simulink model "hibrido_sim"  (R2013a)
settings: Solver=ode3  StartTime=0.0  StopTime=6  FixedStep=Tm  MaxStep=1e-2  RelTol=1e-3
values from neighbouring files (symbols this model uses):
  Ke = 1000    [fuerzas_var.m]    (also in hibrido_var.m)
  Kp = (2*pi*5)^2*eye(3)    [cartesiano_var.m]    (also in hibrido_var.m)
  Kpf = (2*pi*20)^2*eye(3)    [fuerzas_var.m]    (also in hibrido_var.m)
  Kv = 2*sqrt(Kp)*eye(3)    [cartesiano_var.m]    (also in hibrido_var.m)
  Kvf = 2*sqrt(Kpf)*eye(3)    [fuerzas_var.m]    (also in hibrido_var.m)
  q0 = [pi;1/4*pi]    [cartesiano_var.m]    (also in fuerzas_var.m = [0;pi/2]; hibrido_var.m = [0;pi/2])
  R0c = [cX0,cY0,cZ0]    [hibrido_var.m]
  robotTP = robotRR    [cartesiano_var.m]    (also in fuerzas_var.m; hibrido_var.m)
  Sfue = [zeros(1,3);[0,1,0];zeros(1,3)]    [hibrido_var.m]
  Spos = [[1,0,0];zeros(2,3)]    [hibrido_var.m]
  T0c = [R0c,cP0;[0,0,0,1]]    [hibrido_var.m]
undefined symbols (not defined in the file or in its folder): jacob0, modelAlpha, modelBeta
undefined symbols (not defined in the file): robotPlanta
libraries: roblocks x4
settings Model: Creator=Nicola  LastModifiedBy=Nicola

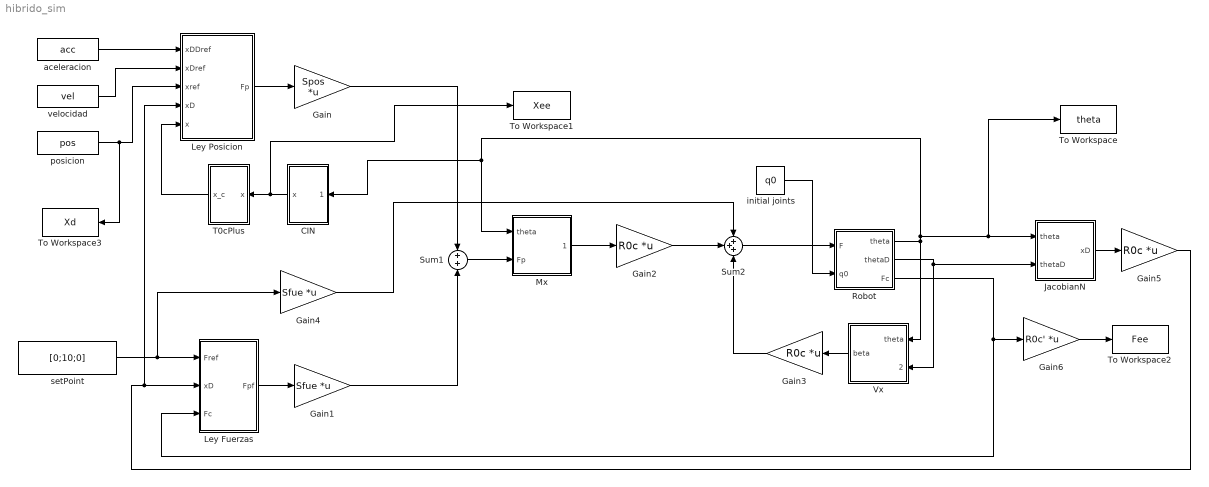
== system hibrido_sim ==
  CIN : Subsystem
  Gain : Gain  Gain=Spos  Multiplication=Matrix(K*u)
  Gain1 : Gain  Gain=Sfue  Multiplication=Matrix(K*u)
  Gain2 : Gain  Gain=R0c  Multiplication=Matrix(K*u)
  Gain3 : Gain  Gain=R0c  Multiplication=Matrix(K*u)
  Gain4 : Gain  Gain=Sfue  Multiplication=Matrix(K*u)
  Gain5 : Gain  Gain=R0c  Multiplication=Matrix(K*u)
  Gain6 : Gain  Gain=R0c'  Multiplication=Matrix(K*u)
  JacobianN : Subsystem
  Ley Fuerzas : Subsystem
  Ley Posicion : Subsystem
  Mx : Subsystem
  Robot : Subsystem
  Sum1 : Sum  Inputs=+|+
  Sum2 : Sum  Inputs=+++
  T0cPlus : Subsystem
  To Workspace : ToWorkspace  VariableName=theta  SampleTime=-1  SaveFormat=Timeseries
  To Workspace1 : ToWorkspace  VariableName=Xee  SampleTime=-1  SaveFormat=Timeseries
  To Workspace2 : ToWorkspace  VariableName=Fee  SampleTime=-1  SaveFormat=Timeseries
  To Workspace3 : ToWorkspace  VariableName=Xd  SampleTime=-1  SaveFormat=Timeseries
  Vx : Subsystem
  aceleracion : FromWorkspace  VariableName=acc  SampleTime=0
  initial joints : Constant  Value=q0
  posicion : FromWorkspace  VariableName=pos  SampleTime=0
  setPoint : Constant  Value=[0;10;0]
  velocidad : FromWorkspace  VariableName=vel  SampleTime=0
  wires:
  aceleracion/1 -> Ley Posicion/1(xDDref)
  velocidad/1 -> Ley Posicion/2(xDref)
  posicion/1 -> To Workspace3/1, Ley Posicion/3(xref)
  Ley Posicion/1(Fp) -> Gain/1
  Gain/1 -> Sum1/1
  setPoint/1 -> Gain4/1, Ley Fuerzas/1(Fref)
  Ley Fuerzas/1(Fpf) -> Gain1/1
  Gain1/1 -> Sum1/2
  Sum1/1 -> Mx/2(Fp)
  Mx/1(Mx*Fp) -> Gain2/1
  Vx/1(beta) -> Gain3/1
  Gain2/1 -> Sum2/2
  Gain3/1 -> Sum2/3
  Gain4/1 -> Sum2/1
  initial joints/1 -> Robot/2(q0)
  Sum2/1 -> Robot/1(F)
  Robot/1(theta) -> Vx/1(theta), To Workspace/1, JacobianN/1(theta), Mx/1(theta), CIN/1(theta)
  Robot/2(thetaD) -> Vx/2(thetaD), JacobianN/2(thetaD)
  Robot/3(Fc) -> Gain6/1, Ley Fuerzas/3(Fc)
  JacobianN/1(xD) -> Gain5/1
  Gain5/1 -> Ley Posicion/4(xD), Ley Fuerzas/2(xD)
  T0cPlus/1(x_c) -> Ley Posicion/5(x)
  CIN/1(x) -> To Workspace1/1, T0cPlus/1(x)
  Gain6/1 -> To Workspace2/1

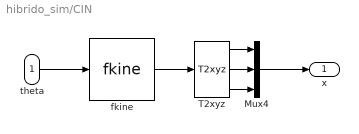
== system hibrido_sim/CIN ==
  theta : Inport
  Mux4 : Mux  Inputs=3
  T2xyz : roblocks/Transform Conversion/T2xyz
  fkine : roblocks/Kinematics/fkine  robot=robotTP.links
  x : Outport
  wires:
  T2xyz/1 -> Mux4/1
  T2xyz/3 -> Mux4/3
  Mux4/1 -> x/1
  T2xyz/2 -> Mux4/2
  theta/1 -> fkine/1
  fkine/1 -> T2xyz/1

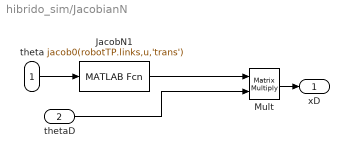
== system hibrido_sim/JacobianN ==
  theta : Inport
  thetaD : Inport  Port=2
  JacobN1 : MATLABFcn  MATLABFcn=jacob0(robotTP.links,u,'trans')  OutputDimensions=[3,2]  Output1D=off
  Mult : Product  Multiplication=Matrix(*)
  xD : Outport
  wires:
  Mult/1 -> xD/1
  thetaD/1 -> Mult/2
  JacobN1/1 -> Mult/1
  theta/1 -> JacobN1/1

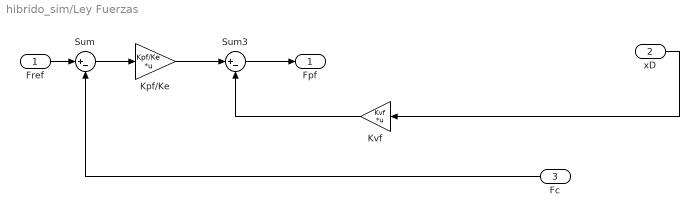
== system hibrido_sim/Ley Fuerzas ==
  Fref : Inport
  xD : Inport  Port=2
  Fc : Inport  Port=3
  Kpf/Ke : Gain  Gain=Kpf/Ke  Multiplication=Matrix(K*u)
  Kvf : Gain  Gain=Kvf  Multiplication=Matrix(K*u)
  Sum : Sum  Inputs=|+-
  Sum3 : Sum  Inputs=|+-
  Fpf : Outport
  wires:
  Fc/1 -> Sum/2
  Sum3/1 -> Fpf/1
  Sum/1 -> Kpf/Ke/1
  Kvf/1 -> Sum3/2
  Kpf/Ke/1 -> Sum3/1
  xD/1 -> Kvf/1
  Fref/1 -> Sum/1

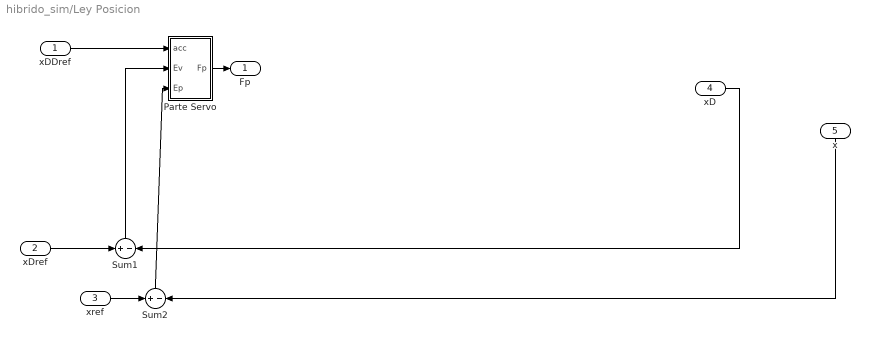
== system hibrido_sim/Ley Posicion ==
  xDDref : Inport
  xDref : Inport  Port=2
  xref : Inport  Port=3
  xD : Inport  Port=4
  x : Inport  Port=5
  Parte Servo : Subsystem
  Sum1 : Sum  Inputs=+|-
  Sum2 : Sum  Inputs=+|-
  Fp : Outport
  wires:
  xDDref/1 -> Parte Servo/1(acc)
  xDref/1 -> Sum1/1
  x/1 -> Sum2/2
  Parte Servo/1(Fp) -> Fp/1
  xref/1 -> Sum2/1
  Sum2/1 -> Parte Servo/3(Ep)
  Sum1/1 -> Parte Servo/2(Ev)
  xD/1 -> Sum1/2

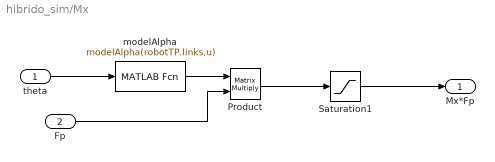
== system hibrido_sim/Mx ==
  theta : Inport
  Fp : Inport  Port=2
  Product : Product  Multiplication=Matrix(*)
  Saturation1 : Saturate  UpperLimit=1e10  LowerLimit=-1e10
  modelAlpha : MATLABFcn  MATLABFcn=modelAlpha(robotTP.links,u)  OutputDimensions=[3,3]  Output1D=off
  Mx*Fp : Outport
  wires:
  modelAlpha/1 -> Product/1
  Fp/1 -> Product/2
  theta/1 -> modelAlpha/1
  Product/1 -> Saturation1/1
  Saturation1/1 -> Mx*Fp/1

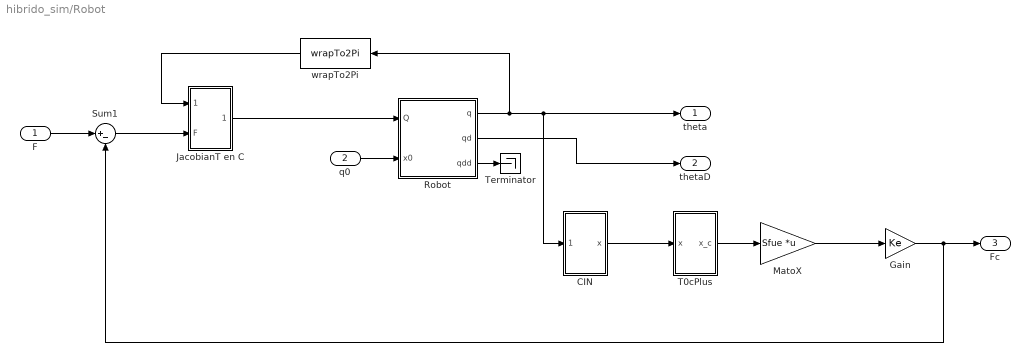
== system hibrido_sim/Robot ==
  F : Inport
  q0 : Inport  Port=2
  CIN : Subsystem
  Gain : Gain  Gain=Ke
  JacobianT en C : Subsystem
  MatoX : Gain  Gain=Sfue  Multiplication=Matrix(K*u)
  Robot : Subsystem  AncestorBlock=roblocks/Dynamics/Robot  mask{robot=robotPlanta, q0=[0,0,0,0,0,0]}
      mask prompts: robot "Robot object"; q0 "Initial state"
      mask help: Rigid-body dynamic model of robot.
      mask init:
      | if isa(robot, 'SerialLink')
      |     rname = robot.name;
      |     %fprintf('**robot name is %s\n', rname);
      | else
      |     rname = '';
      |     n = 0
      | end
      mask Help:
      | Simulates the forward (direct) rigid-body dynamics of the robot described
      | by the given robot object.  For given applied joint torque/force it computes
      | the instaneous joint coordinates, velocities and acclerations.
      | 
      | 
      | <b>Parameters::</b>
      | 
      | robot (SerialLink) a dynamic model of an N-link serial link manipulator
      | q0 (1xN)  Initial joint coordinates
      | 
      | <b>Inputs::</b>
      | 
      | Q (1xN) the generalized joint force (torque or force) required to achieve
      | the motion state (q, qd, qdd).
      | 
      | <b>Outputs::</b>
      | 
      | q (1xN) joint coordinates
      | qd (1xN) joint coordinate velocity
      | qdd (1xN) joint coordinate acceleration
      | 
      | 
      | <b>Notes::</b>
      | 
      | - Required to simulate robot rigid body motion.
      | - Implemented using the recursive Newton-Euler scheme (RNE).
      | - A wrapper for the Toolbox method accel() which in turn depends on the
      |   method rne().
      mask Display:
      | port_label('input', 1, 'Q')
      | port_label('output', 1, 'q')
      | port_label('output', 2, 'qd')
      | port_label('output', 3, 'qdd')
      | text(0.1, 0.9,  rname, 'horizontalAlignment', 'left')
  Sum1 : Sum  Inputs=|+-
  T0cPlus : Subsystem
  Terminator : Terminator
  wrapTo2Pi : MATLABFcn  MATLABFcn=wrapTo2Pi
  theta : Outport
  thetaD : Outport  Port=2
  Fc : Outport  Port=3
  wires:
  Robot/1(q) -> wrapTo2Pi/1, CIN/1(theta), theta/1
  Robot/3(qdd) -> Terminator/1
  Robot/2(qd) -> thetaD/1
  q0/1 -> Robot/2(x0)
  Gain/1 -> Sum1/2, Fc/1
  Sum1/1 -> JacobianT en C/2(F)
  wrapTo2Pi/1 -> JacobianT en C/1(theta)
  F/1 -> Sum1/1
  MatoX/1 -> Gain/1
  T0cPlus/1(x_c) -> MatoX/1
  CIN/1(x) -> T0cPlus/1(x)
  JacobianT en C/1(tau) -> Robot/1(Q)

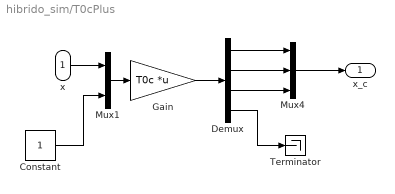
== system hibrido_sim/T0cPlus ==
  x : Inport
  Constant : Constant
  Demux : Demux
  Gain : Gain  Gain=T0c  Multiplication=Matrix(K*u)
  Mux1 : Mux  Inputs=2
  Mux4 : Mux  Inputs=3
  Terminator : Terminator
  x_c : Outport
  wires:
  Mux4/1 -> x_c/1
  Constant/1 -> Mux1/2
  x/1 -> Mux1/1
  Mux1/1 -> Gain/1
  Demux/1 -> Mux4/1
  Demux/2 -> Mux4/2
  Demux/3 -> Mux4/3
  Gain/1 -> Demux/1
  Demux/4 -> Terminator/1

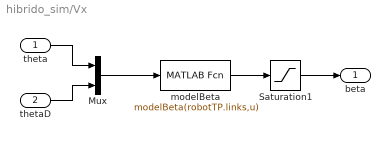
== system hibrido_sim/Vx ==
  theta : Inport
  thetaD : Inport  Port=2
  Mux : Mux  Inputs=2
  Saturation1 : Saturate  UpperLimit=1e3  LowerLimit=-1e3
  modelBeta : MATLABFcn  MATLABFcn=modelBeta(robotTP.links,u)  OutputDimensions=[3,1]  Output1D=off
  beta : Outport
  wires:
  theta/1 -> Mux/1
  thetaD/1 -> Mux/2
  Mux/1 -> modelBeta/1
  modelBeta/1 -> Saturation1/1
  Saturation1/1 -> beta/1

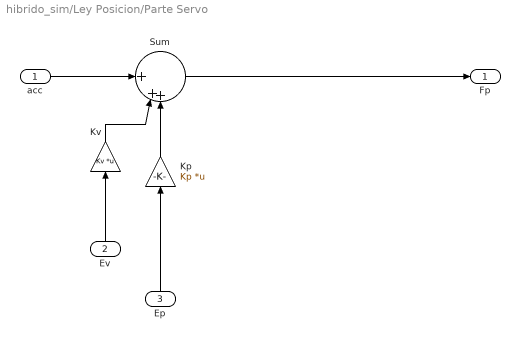
== system hibrido_sim/Ley Posicion/Parte Servo ==
  acc : Inport
  Ev : Inport  Port=2
  Ep : Inport  Port=3
  Kp : Gain  Gain=Kp  Multiplication=Matrix(K*u)
  Kv : Gain  Gain=Kv  Multiplication=Matrix(K*u)
  Sum : Sum  Inputs=||||+||++
  Fp : Outport
  wires:
  acc/1 -> Sum/1
  Ev/1 -> Kv/1
  Kp/1 -> Sum/3
  Ep/1 -> Kp/1
  Kv/1 -> Sum/2
  Sum/1 -> Fp/1

== system hibrido_sim/Robot/CIN ==
  theta : Inport
  Mux4 : Mux  Inputs=3
  T2xyz : roblocks/Transform Conversion/T2xyz
  fkine : roblocks/Kinematics/fkine  robot=robotTP.links
  x : Outport
  wires:
  T2xyz/1 -> Mux4/1
  T2xyz/3 -> Mux4/3
  Mux4/1 -> x/1
  T2xyz/2 -> Mux4/2
  theta/1 -> fkine/1
  fkine/1 -> T2xyz/1

== system hibrido_sim/Robot/JacobianT en C ==
  theta : Inport
  F : Inport  Port=2
  Jacob en C : MATLABFcn  MATLABFcn=jacob0(robotTP.links,u,'trans')'*R0c'  OutputDimensions=[2,3]  Output1D=off
  Product : Product  Multiplication=Matrix(*)
  tau : Outport
  wires:
  theta/1 -> Jacob en C/1
  F/1 -> Product/2
  Product/1 -> tau/1
  Jacob en C/1 -> Product/1

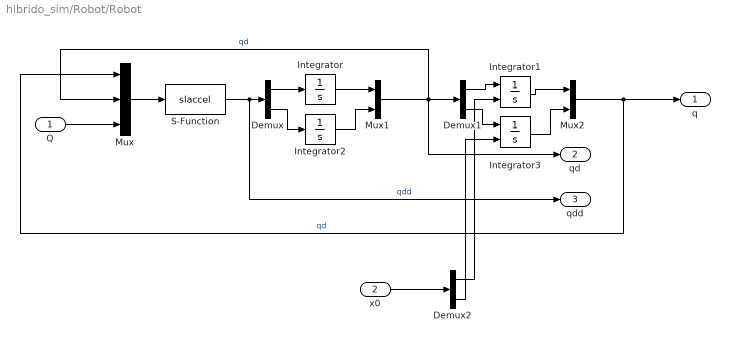
== system hibrido_sim/Robot/Robot ==
  Q : Inport
  x0 : Inport  Port=2
  Demux : Demux  Outputs=2
  Demux1 : Demux  Outputs=2
  Demux2 : Demux  Outputs=2
  Integrator : Integrator
  Integrator1 : Integrator  InitialConditionSource=external
  Integrator2 : Integrator
  Integrator3 : Integrator  InitialConditionSource=external  InitialCondition=3/4*pi
  Mux : Mux  Inputs=3
  Mux1 : Mux  Inputs=2
  Mux2 : Mux  Inputs=2
  S-Function : S-Function  FunctionName=slaccel  Parameters=robot  EnableBusSupport=off
  q : Outport
  qd : Outport  Port=2
  qdd : Outport  Port=3
  wires:
  Q/1 -> Mux/3
  Mux/1 -> S-Function/1
  S-Function/1 -> Demux/1, qdd/1  "qdd"
  Demux/2 -> Integrator2/1
  Demux/1 -> Integrator/1
  Integrator/1 -> Mux1/1
  Integrator2/1 -> Mux1/2
  Mux1/1 -> Demux1/1, qd/1, Mux/2  "qd"
  Demux1/2 -> Integrator3/1
  Demux1/1 -> Integrator1/1
  Integrator1/1 -> Mux2/1
  Integrator3/1 -> Mux2/2
  Mux2/1 -> Mux/1, q/1  "qd"
  x0/1 -> Demux2/1
  Demux2/1 -> Integrator1/2
  Demux2/2 -> Integrator3/2

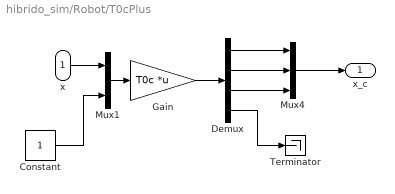
== system hibrido_sim/Robot/T0cPlus ==
  x : Inport
  Constant : Constant
  Demux : Demux
  Gain : Gain  Gain=T0c  Multiplication=Matrix(K*u)
  Mux1 : Mux  Inputs=2
  Mux4 : Mux  Inputs=3
  Terminator : Terminator
  x_c : Outport
  wires:
  Mux4/1 -> x_c/1
  Constant/1 -> Mux1/2
  x/1 -> Mux1/1
  Mux1/1 -> Gain/1
  Demux/1 -> Mux4/1
  Demux/2 -> Mux4/2
  Demux/3 -> Mux4/3
  Gain/1 -> Demux/1
  Demux/4 -> Terminator/1
